simulink model "SomanetConfigHandler"  (R2016b)
settings: Solver=FixedStepDiscrete  StartTime=0.0  StopTime=inf  RelTol=1e-3  EnableMultiTasking=on
settings Model: xpc_rtwmakecfg_data=_xpcethercatlib_  Creator=march  LastModifiedBy=march
settings SolverCC: EnableConcurrentExecution=on  AutoInsertRateTranBlk=on
settings DataIOCC: SaveFormat=StructureWithTime  SaveOutput=off  SaveTime=off
settings OptimizationCC: BlockReduction=off  OptimizeBlockIOStorage=off  BufferReuse=off  GlobalBufferReuse=off  ExpressionFolding=off  LocalBlockOutputs=off
settings HardwareCC: ProdBitPerPointer=32  ProdBitPerSizeT=32  ProdBitPerPtrDiffT=32  ProdLargestAtomicFloat=None  ProdWordSize=32  ProdLongLongMode=on  ProdHWDeviceType=Generic->32-bit x86 compatible
settings RTWCC: SystemTargetFile=slrt.tlc  TemplateMakefile=slrt_default_tmf  PostCodeGenCommand=SomanetTuning_make_rtw_hook  Description=Simulink Real-Time  RTWVerbose=off  CodeExecutionProfiling=on  RTWCompilerOptimization=on
settings SimulinkRealTimeCC: xPCModelTimeoutSecs=20

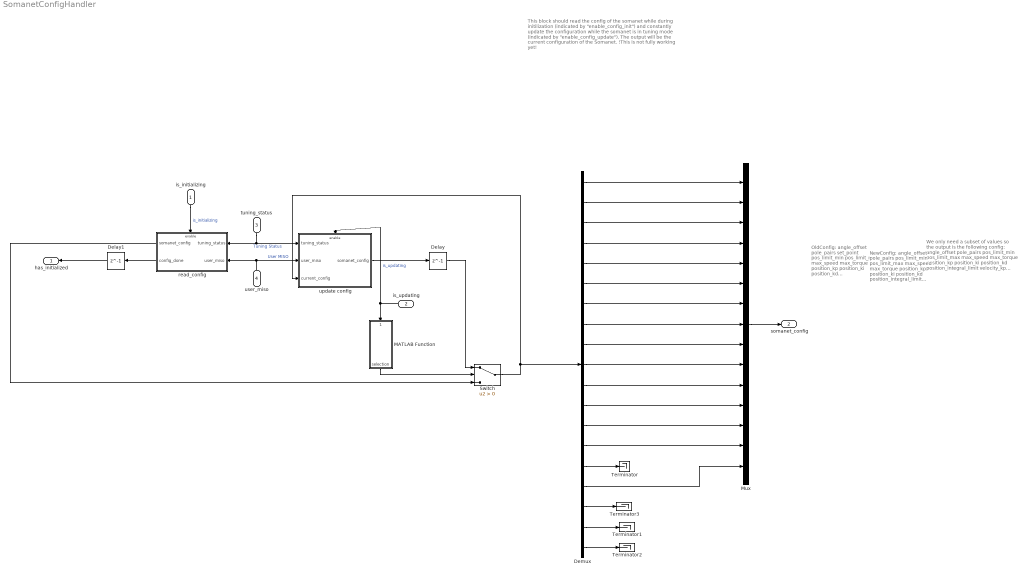
== system SomanetConfigHandler ==
  note: OldConfig:
      | angle_offset
      | pole_pairs
      | set_point
      | pos_limit_min
      | pos_limit_max
      | max_speed
      | max_torque
      | position_kp
      | position_ki
      | position_kd
      | position_integral_limit
      | velocity_kp
      | velocity_ki
      | velocity_kd
      | velocity_integral_limit
      | error_status
      | break_release_strategy
      | sensor_error
  note: This block should read the config of the somanet while
      | during initilization (indicated by "enable_config_init") and
      | constantly update the configuration while the somanet
      | is in tuning mode (indicated by "enable_config_update").
      | The output will be the current configuration of the Somanet.
      | !This is not fully working yet!
  note: We only need a subset of values
      | so the output is the following config:
      | angle_offset
      | pole_pairs
      | pos_limit_min
      | pos_limit_max
      | max_speed
      | max_torque
      | position_kp
      | position_ki
      | position_kd
      | position_integral_limit
      | velocity_kp
      | velocity_ki
      | velocity_kd
      | velocity_integral_limit
      | break_release_strategy
  note: NewConfig:
      | angle_offset
      | pole_pairs
      | pos_limit_min
      | pos_limit_max
      | max_speed
      | max_torque
      | position_kp
      | position_ki
      | position_kd
      | position_integral_limit
      | velocity_kp
      | velocity_ki
      | velocity_kd
      | velocity_integral_limit
      | error_status
      | break_release_strategy
      | sensor_error
      | motion_control_error
      | rated_torque
  is_initializing : Inport  OutDataTypeStr=boolean  PortDimensions=1  SampleTime=[0.002,0]
  is_updating : Inport  Port=2  OutDataTypeStr=boolean  PortDimensions=1  SampleTime=[0.002,0]
  tuning_status : Inport  Port=3  OutDataTypeStr=uint32  PortDimensions=1  SampleTime=[0.002,0]
  user_miso : Inport  Port=4  OutDataTypeStr=uint32  PortDimensions=1  SampleTime=[0.002,0]
  Delay : Delay  DelayLength=1
  Delay1 : Delay  DelayLength=1
  Demux : Demux  Outputs=19
  MATLAB Function : MATLAB Function  TreatAsAtomicUnit=on
  Mux : Mux  Inputs=15
  Switch : Switch  Criteria=u2 > Threshold
  Terminator{,1..3} (4 alike) : Terminator
  read_config : Subsystem  TreatAsAtomicUnit=on
  update config : Subsystem  TreatAsAtomicUnit=on
  has_initialized : Outport  OutDataTypeStr=boolean  PortDimensions=1  SampleTime=[0.002,0]
  somanet_config : Outport  Port=2  OutDataTypeStr=double  PortDimensions=15  SampleTime=[0.002,0]
  wires:
  update config/1(somanet_config) -> Delay/1
  tuning_status/1 -> update config/1(tuning_status), read_config/1(tuning_status)  "Tuning Status"
  user_miso/1 -> update config/2(user_miso), read_config/2(user_miso)  "User MISO"
  Switch/1 -> Demux/1, update config/3(current_config)
  read_config/2(config_done) -> Delay1/1
  is_initializing/1 -> read_config/Enable  "is_initializing"
  Delay1/1 -> has_initialized/1
  read_config/1(somanet_config) -> Switch/3
  Delay/1 -> Switch/1
  Mux/1 -> somanet_config/1
  Demux/2 -> Mux/2
  MATLAB Function/1(selection) -> Switch/2
  Demux/1 -> Mux/1
  Demux/18 -> Terminator1/1
  Demux/3 -> Mux/3
  is_updating/1 -> update config/Enable, MATLAB Function/1(enable_config_update)  "is_updating"
  Demux/4 -> Mux/4
  Demux/5 -> Mux/5
  Demux/6 -> Mux/6
  Demux/7 -> Mux/7
  Demux/8 -> Mux/8
  Demux/9 -> Mux/9
  Demux/10 -> Mux/10
  Demux/11 -> Mux/11
  Demux/12 -> Mux/12
  Demux/13 -> Mux/13
  Demux/14 -> Mux/14
  Demux/15 -> Terminator/1
  Demux/16 -> Mux/15
  Demux/17 -> Terminator3/1
  Demux/19 -> Terminator2/1

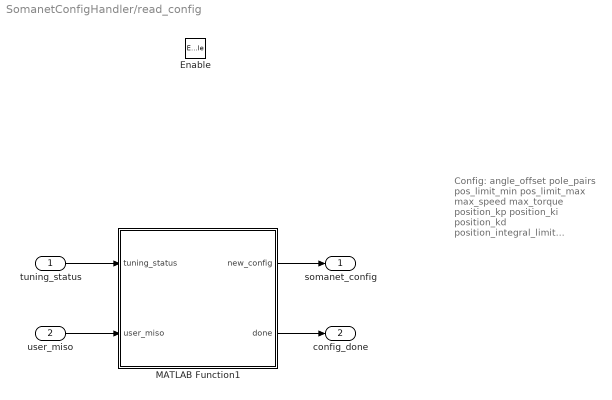
== system SomanetConfigHandler/read_config ==
  note: Config:
      | angle_offset
      | pole_pairs
      | pos_limit_min
      | pos_limit_max
      | max_speed
      | max_torque
      | position_kp
      | position_ki
      | position_kd
      | position_integral_limit
      | velocity_kp
      | velocity_ki
      | velocity_kd
      | velocity_integral_limit
      | error_status
      | break_release_strategy
      | sensor_error
      | motion_control_error
      | rated_torque
  tuning_status : Inport
  user_miso : Inport  Port=2
  Enable : EnablePort
  MATLAB Function1 : MATLAB Function  TreatAsAtomicUnit=on
  somanet_config : Outport
  config_done : Outport  Port=2
  wires:
  user_miso/1 -> MATLAB Function1/2(user_miso)
  tuning_status/1 -> MATLAB Function1/1(tuning_status)
  MATLAB Function1/2(done) -> config_done/1
  MATLAB Function1/1(new_config) -> somanet_config/1

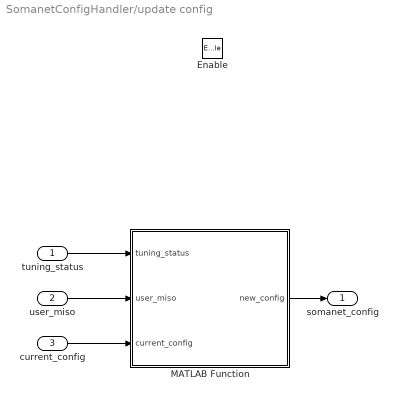
== system SomanetConfigHandler/update config ==
  tuning_status : Inport
  user_miso : Inport  Port=2
  current_config : Inport  Port=3
  Enable : EnablePort
  MATLAB Function : MATLAB Function  TreatAsAtomicUnit=on
  somanet_config : Outport
  wires:
  user_miso/1 -> MATLAB Function/2(user_miso)
  MATLAB Function/1(new_config) -> somanet_config/1
  current_config/1 -> MATLAB Function/3(current_config)
  tuning_status/1 -> MATLAB Function/1(tuning_status)

== matlab function SomanetConfigHandler/read_config/MATLAB Function1 ==
  data: tuning_status input; new_config output int32; user_miso input; done output
function [new_config,done] = read_config(tuning_status,user_miso)
    persistent calls;
    persistent buffered_config;
    N_params = 19;
    if(isempty(calls))
        calls = 0;
        buffered_config = zeros(N_params,1);
    end
  
    
    status_mux = bitand(bitsra(tuning_status,16),hex2dec('FF'));
   
    if status_mux <= N_params && status_mux >= 1
        calls = calls + 1;
        buffered_config(status_mux) = user_miso;
        %TODO error handling here?
    end
    
    if calls > N_params + 10 % we might want to increase this. We have noticed that sometimes an important value like maxpos does not get properly initalized and instead is zero
        done = true;
    else
        done = false;
    end
    
    new_config = to_signed_int32(buffered_config);
end

== matlab function SomanetConfigHandler/update config/MATLAB Function ==
  data: tuning_status input; new_config output; user_miso input; current_config input
function new_config = update_config(tuning_status,user_miso,current_config)
    status_mux = bitand(bitsra(tuning_status,16),hex2dec('FF'));
    N_params = 19;
    
    new_config = current_config;
    if status_mux <= N_params
        new_config(status_mux) = to_signed_int32(user_miso);
        %TODO error handling here?
    end

== matlab function SomanetConfigHandler/MATLAB Function ==
  data: enable_config_update input; selection output
function selection = select_config_loop(enable_config_update)
%% Selects whether to output values from read_config or from update_config
% Once update_config has run once, that config stores the correct values
% So, after going back to cyclic operation from tuning mode, update_config
% outputs the correct config even though it's not running
% Therefore: if enable_config_update was true ever, always pick the values
% from update_config

persistent post_init;
if isempty(post_init)
    post_init = false;
end
post_init = or(post_init, enable_config_update);
selection = post_init;
end
